simulink model "Lab5_Ris_2_15"  (Simulink 10.2)
settings: Solver=VariableStepAuto  StartTime=0.0  StopTime=12  RelTol=1e-3
libraries: commsequence2 x1, commseqgen3 x1, commutil2 x1
settings Model: Creator=Newtr  LastModifiedBy=Newtr
settings DataIOCC: SaveFormat=Dataset  SignalLoggingSaveFormat=Dataset  ReturnWorkspaceOutputs=on
settings OptimizationCC: LifeSpan=auto
settings DebuggingCC: UnderspecifiedInitializationDetection=Simplified  MergeDetectMultiDrivingBlocksExec=error  FcnCallInpInsideContextMsg=error  SFUnexpectedBacktrackingDiag=error  SFNoUnconditionalDefaultTransitionDiag=error  SFExecutionAtInitializationDiag=warning  ArithmeticOperatorsInVariantConditions=error
settings HardwareCC: ProdBitPerPointer=64  ProdBitPerSizeT=64  ProdBitPerPtrDiffT=64  ProdLargestAtomicFloat=Float  ProdIntDivRoundTo=Zero  ProdEndianess=LittleEndian  ProdWordSize=64  ProdHWDeviceType=Intel->x86-64 (Windows64)
settings ModelReferenceCC: PropagateSignalLabelsOutOfModel=on
settings SFSimCC: SimUseLocalCustomCode=on  CustomCodeUndefinedFunction=FilterOut
settings RTWCC: RTWUseLocalCustomCode=on
settings CodeAppCC: StateflowObjectComments=off
settings GRTTargetCC: TargetLangStandard=C99 (ISO)  CombineOutputUpdateFcns=on  GRTInterface=off
settings ConfigComp: CovMetricSettings=dwe  CovSaveCumulativeToWorkspaceVar=off  CovSaveSingleToWorkspaceVar=off  CovExternalEMLEnable=on

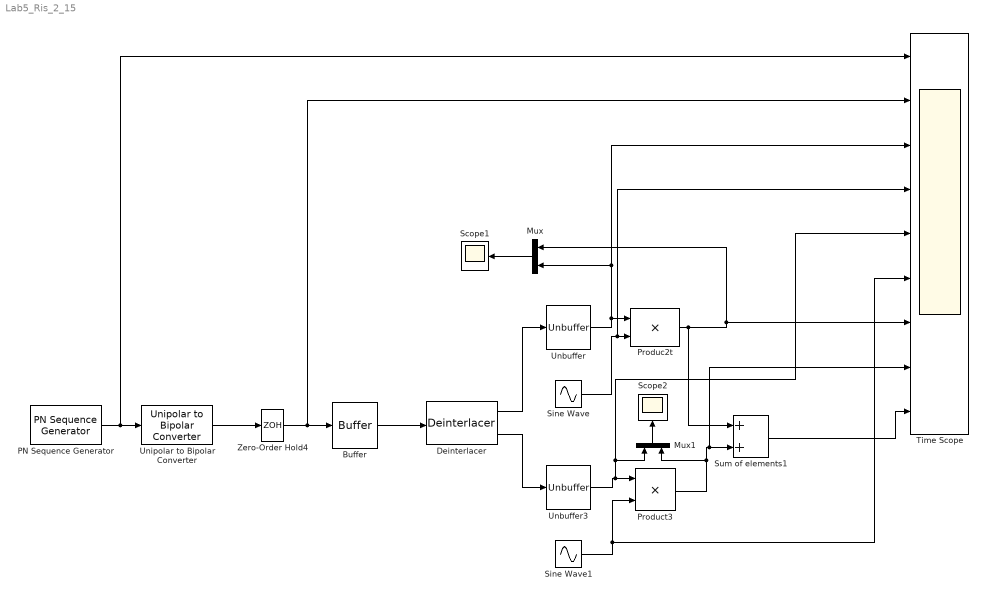
== system Lab5_Ris_2_15 ==
  Buffer : Buffer  N=2  OutputFrames=off
  Deinterlacer : commsequence2/Deinterlacer
      settings: SourceProductBaseCode=CM
  Mux : Mux  Inputs=2
  Mux1 : Mux  Inputs=2
  PN Sequence Generator : commseqgen3/PN Sequence Generator  poly='z^6 + z + 1'  ini_sta=[0 0 0 0 0 1]  outBitMaskSource=Dialog parameter  shift=0  outVarSiz=off  maxOutSizeMode=Dialog parameter  maxOutSize=[10 1]  Ts=1/1200  sampPerFrame=1  reset=off  bitPackedOutputs=off  outDataType=double  numPackedBits=8  bitPackDataSigned=off  bitPackedOutDType=double
  Produc2t : Product
  Product3 : Product
  Scope1 : Scope
  Scope2 : Scope
  Sine Wave : Sin  Frequency=753600  Phase=-pi/2  SampleTime=0
  Sine Wave1 : Sin  Frequency=753600  SampleTime=0
  Sum of elements1 : Sum
  Time Scope : Scope  NumInputPorts=9
  Unbuffer : Unbuffer
  Unbuffer3 : Unbuffer
  Unipolar to Bipolar Converter : commutil2/Unipolar to Bipolar Converter  M=2  polarity=Positive  dataType=Inherit via internal rule
  Zero-Order Hold4 : ZeroOrderHold  SampleTime=-1
  wires:
  PN Sequence Generator/1 -> Time Scope/1, Unipolar to Bipolar Converter/1
  Unipolar to Bipolar Converter/1 -> Zero-Order Hold4/1
  Zero-Order Hold4/1 -> Time Scope/2, Buffer/1
  Buffer/1 -> Deinterlacer/1
  Deinterlacer/1 -> Unbuffer/1
  Deinterlacer/2 -> Unbuffer3/1
  Sine Wave1/1 -> Time Scope/6, Product3/2
  Unbuffer3/1 -> Time Scope/5, Mux1/1, Product3/1
  Product3/1 -> Mux1/2, Time Scope/8, Sum of elements1/2
  Sum of elements1/1 -> Time Scope/9
  Mux1/1 -> Scope2/1
  Unbuffer/1 -> Time Scope/3, Mux/2, Produc2t/1
  Produc2t/1 -> Sum of elements1/1, Time Scope/7, Mux/1
  Sine Wave/1 -> Time Scope/4, Produc2t/2
  Mux/1 -> Scope1/1
